simulink model "gm_ADC_personal"  (R2024a)
settings: Solver=FixedStepAuto  StartTime=0.0  StopTime=600e-06  FixedStep=1/250e6  RelTol=1e-3
PreLoadFcn:
  | jitter = 145e-15;
  | nonlingain = 0.17;
StopFcn:
  | dy = out.yout - mean(out.yout);
  | rmsjitter = std(dy);
  | histogram(dy,50);
  | title(['\bfjitter didtribution: RMS jitter = ',num2str(rmsjitter),'s']);
  | xlabel('Time (s) -->');
  | ylabel('Occurances (count) -->');
libraries: dspfdesign x2, hdlmdlgenlib x1
settings Model: Creator=GILBERT KELECHI  LastModifiedBy=GILBERT KELECHI
settings DataIOCC: LimitDataPoints=on  MaxDataPoints=200000  SaveFormat=Array
settings OptimizationCC: BlockReduction=off  ConditionallyExecuteInputs=off
settings DebuggingCC: InheritedTsInSrcMsg=none  SingleTaskRateTransMsg=error
settings HardwareCC: ProdBitPerPointer=32  ProdBitPerSizeT=32  ProdBitPerPtrDiffT=32  ProdLargestAtomicFloat=None  ProdWordSize=32  ProdHWDeviceType=Altera->SoC (ARM Cortex A)  TargetBitPerPointer=64  TargetBitPerSizeT=64  TargetBitPerPtrDiffT=64  TargetLongLongMode=on  TargetIntDivRoundTo=Zero  TargetEndianess=LittleEndian  TargetWordSize=64  TargetHWDeviceType=Custom Processor->MATLAB Host Computer  ProdEqTarget=off
settings RTWCC: GenCodeOnly=on

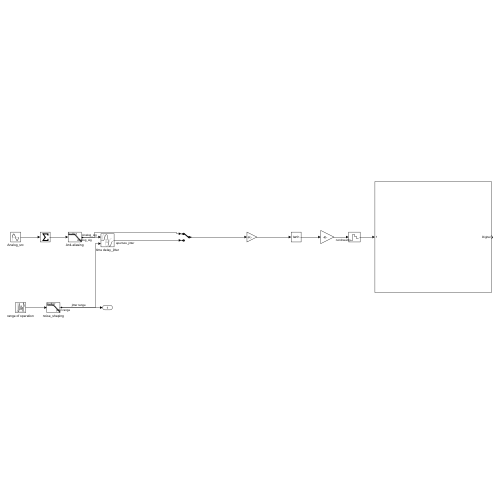
[thumbnail: Simulink's stored preview of the top-level diagram]
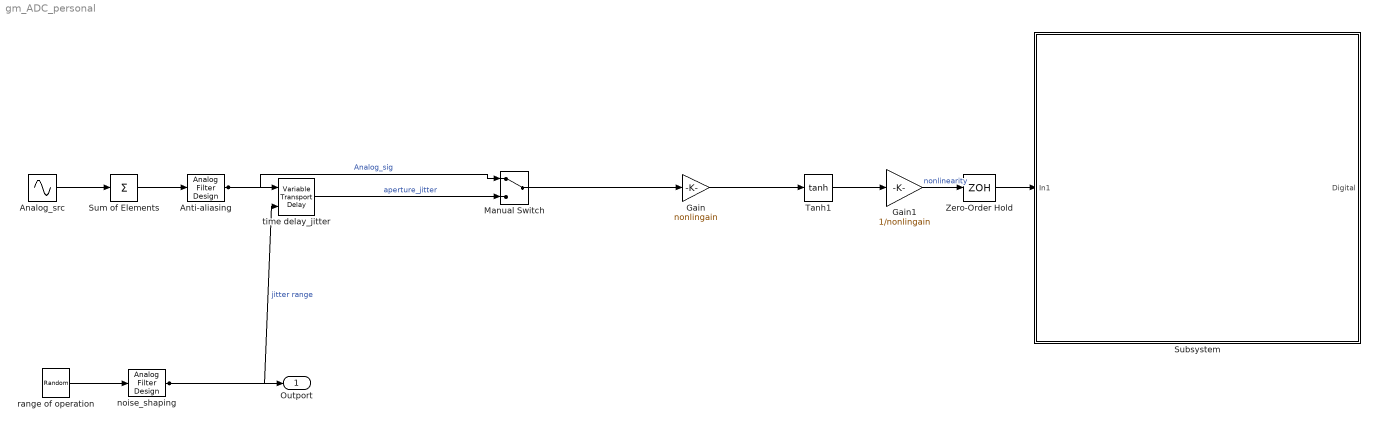
== system gm_ADC_personal ==
  Analog_src : Sin  Amplitude=0.5  Frequency=2*pi*20e6  SampleTime=0
  Anti-aliasing : dspfdesign/Analog Filter Design  method=Butterworth  filttype=Lowpass  N=8  Wlo=2*pi*125e6  Whi=80  Rp=2  Rs=40
  Gain : Gain  Gain=nonlingain
  Gain1 : Gain  Gain=1/nonlingain
  Manual Switch : ManualSwitch
  Subsystem : Subsystem
  Sum of Elements : Sum  Inputs=+
  Tanh1 : Trigonometry  Operator=tanh
  Zero-Order Hold : ZeroOrderHold  SampleTime=1/250e6
  noise_shaping : dspfdesign/Analog Filter Design  method=Butterworth  filttype=Lowpass  N=3  Wlo=2*pi*20e6  Whi=80  Rp=2  Rs=40
  range of operation : UniformRandomNumber  Minimum=0  Maximum=10.36*sqrt(12)*jitter  Seed=1234  SampleTime=0
  time delay_jitter : VariableTransportDelay  MaximumDelay=10e-12  ZeroDelay=on  TransDelayFeedthrough=on
  Outport : Outport
  wires:
  Zero-Order Hold/1 -> Subsystem/1(In1)
  Gain1/1 -> Zero-Order Hold/1  "nonlinearity"
  Manual Switch/1 -> Gain/1
  Tanh1/1 -> Gain1/1
  Gain/1 -> Tanh1/1
  Anti-aliasing/1 -> time delay_jitter/1, Manual Switch/1  "Analog_sig"
  Sum of Elements/1 -> Anti-aliasing/1
  time delay_jitter/1 -> Manual Switch/2  "aperture_jitter"
  noise_shaping/1 -> time delay_jitter/2, Outport/1  "jitter range"
  range of operation/1 -> noise_shaping/1
  Analog_src/1 -> Sum of Elements/1

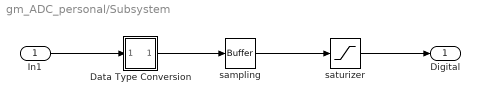
== system gm_ADC_personal/Subsystem ==
  In1 : Inport  OutDataTypeStr=double  PortDimensions=1  SampleTime=4e-09
  Data Type Conversion : Subsystem
      mask Display: disp('NFP\nconv');
  sampling : hdlmdlgenlib/Buffer
  saturizer : Saturate  UpperLimit="fi(0,1,16,14,\"hex\",\"2000\")"  LowerLimit="fi(0,1,16,14,\"hex\",\"e000\")"  SampleTime=4e-09  OutDataTypeStr=fixdt(1, 16, 14)
  Digital : Outport  SampleTime=4e-09
  wires:
  In1/1 -> Data Type Conversion/1(In1)
  sampling/1 -> saturizer/1
  saturizer/1 -> Digital/1
  Data Type Conversion/1(Out1) -> sampling/1

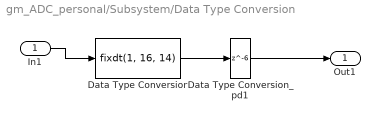
== system gm_ADC_personal/Subsystem/Data Type Conversion ==
  In1 : Inport
  Data Type Conversion : DataTypeConversion  OutDataTypeStr=fixdt(1, 16, 14)  SampleTime=4e-09  SaturateOnIntegerOverflow=off  RndMeth=Floor
  Data Type Conversion_pd1 : Delay  DelayLength=6
  Out1 : Outport
  wires:
  In1/1 -> Data Type Conversion/1
  Data Type Conversion/1 -> Data Type Conversion_pd1/1
  Data Type Conversion_pd1/1 -> Out1/1
